simulink model "Motor_Monitor"  (R2025b)
settings: Solver=VariableStepAuto  StartTime=0.0  StopTime=100  RelTol=1e-3
libraries: simulink x9
settings Model: Creator=abirp  LastModifiedBy=abirp

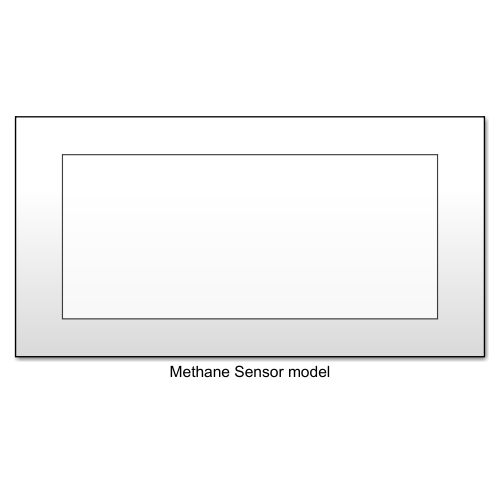
[thumbnail: Simulink's stored preview of the top-level diagram]
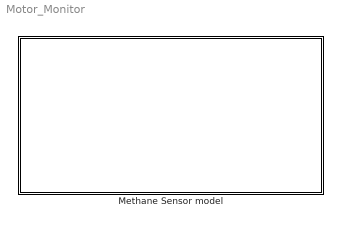
== system Motor_Monitor ==
  Methane Sensor model : Subsystem

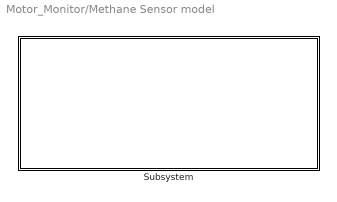
== system Motor_Monitor/Methane Sensor model ==
  Subsystem : Subsystem

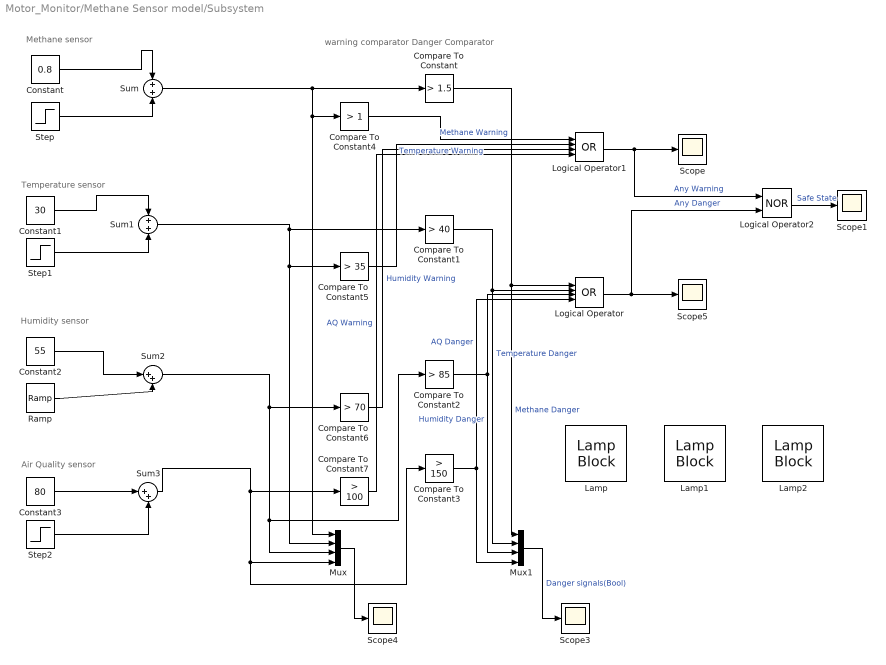
== system Motor_Monitor/Methane Sensor model/Subsystem ==
  note: Danger
      | Comparator
  note: warning
      | comparator
  note: Air Quality sensor
  note: Humidity sensor
  note: Methane sensor
  note: Temperature sensor
  Compare To Constant : simulink/Logic and Bit Operations/Compare To Constant  relop=>  const=1.5  OutDataTypeStr=boolean
  Compare To Constant1 : simulink/Logic and Bit Operations/Compare To Constant  relop=>  const=40  OutDataTypeStr=boolean
  Compare To Constant2 : simulink/Logic and Bit Operations/Compare To Constant  relop=>  const=85  OutDataTypeStr=boolean
  Compare To Constant3 : simulink/Logic and Bit Operations/Compare To Constant  relop=>  const=150  OutDataTypeStr=boolean
  Compare To Constant4 : simulink/Logic and Bit Operations/Compare To Constant  relop=>  const=1  OutDataTypeStr=boolean
  Compare To Constant5 : simulink/Logic and Bit Operations/Compare To Constant  relop=>  const=35  OutDataTypeStr=boolean
  Compare To Constant6 : simulink/Logic and Bit Operations/Compare To Constant  relop=>  const=70  OutDataTypeStr=boolean
  Compare To Constant7 : simulink/Logic and Bit Operations/Compare To Constant  relop=>  const=100  OutDataTypeStr=boolean
  Constant : Constant  Value=0.8
  Constant1 : Constant  Value=30
  Constant2 : Constant  Value=55
  Constant3 : Constant  Value=80
  Lamp : LampBlock  LabelPosition=Hide  DefaultColor=[192.0, 192.0, 192.0]
  Lamp1 : LampBlock  LabelPosition=Hide  DefaultColor=[192.0, 192.0, 192.0]
  Lamp2 : LampBlock  LabelPosition=Hide  DefaultColor=[192.0, 192.0, 192.0]
  Logical Operator : Logic  Operator=OR  Inputs=4  AllPortsSameDT=off  OutDataTypeStr=boolean
  Logical Operator1 : Logic  Operator=OR  Inputs=4  AllPortsSameDT=off  OutDataTypeStr=boolean
  Logical Operator2 : Logic  Operator=NOR  AllPortsSameDT=off  OutDataTypeStr=boolean
  Mux : Mux
  Mux1 : Mux
  Ramp : simulink/Sources/Ramp  slope=1  start=12  InitialOutput=0
  Scope{,1,3..5} (5 alike) : Scope
      Scope settings: ActiveDisplayYMinimum=-1  ActiveDisplayYMaximum=1
      Scope1 settings: ActiveDisplayYMinimum=-0.36048165464550186  ActiveDisplayYMaximum=1.5974443259868876
      Scope3 settings: ActiveDisplayYMinimum=-0.853078770483036  ActiveDisplayYMaximum=1.7521966356215808  DataLoggingVariableName=ScopeData3
      Scope4 settings: ActiveDisplayYMinimum=-20.349999999999998  ActiveDisplayYMaximum=191.15  DataLoggingVariableName=ScopeData4
      Scope5 settings: ActiveDisplayYMinimum=0.675  ActiveDisplayYMaximum=1.9249999999999998  DataLoggingVariableName=ScopeData5
  Step : Step  Time=20  After=0.4  SampleTime=0
  Step1 : Step  Time=15  After=12  OutDataTypeStr=Inherit: Inherit via back propagation  SampleTime=0
  Step2 : Step  Time=20  After=90  SampleTime=0
  Sum : Sum
  Sum1 : Sum
  Sum2 : Sum  Inputs=|++
  Sum3 : Sum  Inputs=|++
  wires:
  Step/1 -> Sum/2
  Constant/1 -> Sum/1
  Sum1/1 -> Compare To Constant5/1, Mux/2, Compare To Constant1/1
  Constant1/1 -> Sum1/1
  Step1/1 -> Sum1/2
  Sum2/1 -> Compare To Constant2/1, Mux/3, Compare To Constant6/1
  Constant2/1 -> Sum2/1
  Ramp/1 -> Sum2/2
  Constant3/1 -> Sum3/1
  Step2/1 -> Sum3/2
  Sum3/1 -> Compare To Constant3/1, Mux/4, Compare To Constant7/1
  Sum/1 -> Compare To Constant4/1, Mux/1, Compare To Constant/1
  Mux/1 -> Scope4/1
  Compare To Constant/1 -> Mux1/1, Logical Operator/1  "Methane Danger"
  Compare To Constant1/1 -> Mux1/2, Logical Operator/2  "Temperature Danger"
  Compare To Constant2/1 -> Mux1/3, Logical Operator/3  "Humidity Danger"
  Compare To Constant3/1 -> Logical Operator/4, Mux1/4  "AQ Danger"
  Logical Operator/1 -> Logical Operator2/2, Scope5/1  "Any Danger"
  Mux1/1 -> Scope3/1  "Danger signals(Bool)"
  Compare To Constant4/1 -> Logical Operator1/1  "Methane Warning"
  Compare To Constant5/1 -> Logical Operator1/2  "Temperature Warning"
  Compare To Constant6/1 -> Logical Operator1/3  "Humidity Warning"
  Compare To Constant7/1 -> Logical Operator1/4  "AQ Warning"
  Logical Operator1/1 -> Logical Operator2/1, Scope/1  "Any Warning"
  Logical Operator2/1 -> Scope1/1  "Safe State"
